simulink model "Bouclage_L"  (R2018b)
settings: Solver=ode45  StartTime=0.0  StopTime=10.0  RelTol=1e-4  EnableMultiTasking=on
values from neighbouring files (symbols this model uses):
  A_nl = [0  0                    1                  0 ;            0  0                    0                  1 ;            0  Ks/Jp                -Phi^2*N^2/(R*Jp)  0 ;            0  -Ks*(Jp+Jb)/(Jp*Jb)  Phi^2*N^2/(R*Jp)   0]    [Script_TP1.m]
  B_nl = [B B_b]    [Script_TP1.m]
  beta = R*Jp*Jb/(Ks*N*Phi)    (= 3.72670807453e-05)    [Script_TP1.m]
  C = [1,  1,  0,  0]    [Script_TP1.m]
  Jb = 0.0059    [Script_TP1.m]
  Ks = 1.61    [Script_TP1.m]
  L = [0, -Ks^2*(Jp+Jb)/(Jp*Jb^2) , Ks*Phi^2*N^2/(R*Jp*Jb), 0]    [Script_TP1.m]
  l1 = m*g*h/Jb    (= 40.1633898305)    [Script_TP1.m]
  l2 = -(m*g*h)^2/(Jb*Jb)    (= -1613.09788268)    [Script_TP1.m]
  l3 = Ks*m*g*h/(Jb^2)    (= 10959.8402758)    [Script_TP1.m]
  l4 = Ks*m*g*h/(Jb*Jb)    (= 10959.8402758)    [Script_TP1.m]
  Somme = [1 1 1 1 1]    [Script_TP1.m]
libraries: simulink x1
settings Model: Creator=abbasturki  LastModifiedBy=pac
settings DataIOCC: LimitDataPoints=on  SaveFormat=Array
settings OptimizationCC: ExpressionDepthLimit=2147483647  LifeSpan=inf
settings DebuggingCC: UnderspecifiedInitializationDetection=Classic  MergeDetectMultiDrivingBlocksExec=none  SolverPrmCheckMsg=warning  StateNameClashWarn=warning  SFUnexpectedBacktrackingDiag=warning  SFNoUnconditionalDefaultTransitionDiag=warning  SFExecutionAtInitializationDiag=none
settings HardwareCC: ProdBitPerPointer=32  ProdBitPerSizeT=32  ProdBitPerPtrDiffT=32  ProdLargestAtomicFloat=None  ProdIntDivRoundTo=Undefined  ProdEndianess=Unspecified  ProdWordSize=32  ProdHWDeviceType=32-bit Generic
settings ModelReferenceCC: PropagateSignalLabelsOutOfModel=off
settings SFSimCC: SimUseLocalCustomCode=off
settings RTWCC: RTWUseLocalCustomCode=off
settings CodeAppCC: StateflowObjectComments=on
settings GRTTargetCC: TargetLangStandard=C89/C90 (ANSI)  GeneratePreprocessorConditionals=Disable all  CombineOutputUpdateFcns=off  GRTInterface=on
settings ConfigComp: CovMetricSettings=dw  CovHtmlReporting=on  CovSaveCumulativeToWorkspaceVar=on  CovSaveSingleToWorkspaceVar=on  CovExternalEMLEnable=off

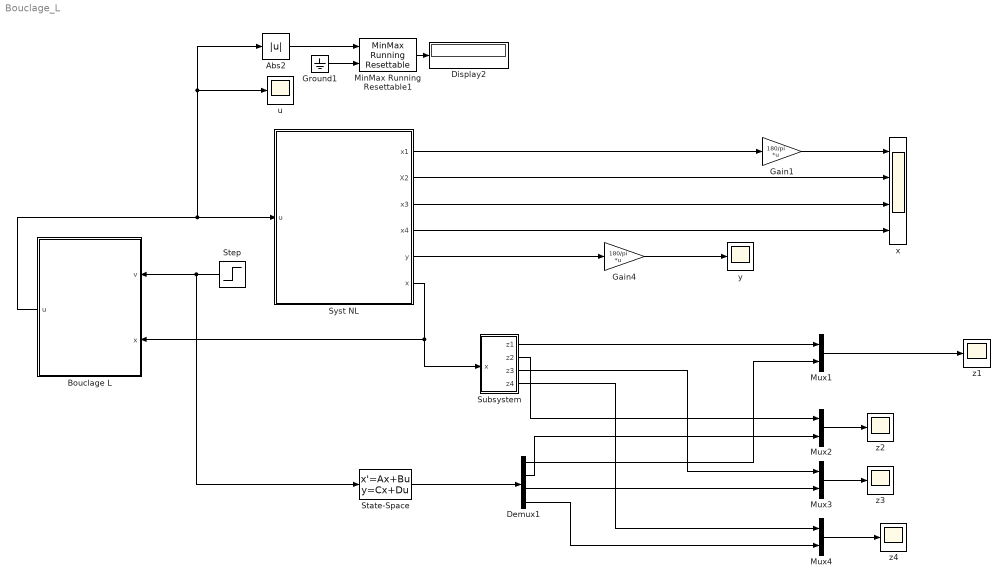
== system Bouclage_L ==
  Abs2 : Abs
  Bouclage L : Subsystem
  Demux1 : Demux
  Display2 : Display
  Gain1 : Gain  Gain=180/pi  Multiplication=Matrix(K*u)
  Gain4 : Gain  Gain=180/pi  Multiplication=Matrix(K*u)
  Ground1 : Ground
  MinMax Running Resettable1 : simulink/Math Operations/MinMax Running Resettable  Function=max  vinit=0.0
  Mux{1..4} (4 alike) : Mux  Inputs=2
  State-Space : StateSpace  A=[0 1 0 0; 0 0 1 0; 0 0 0 1; 0 0 0 0]  B=[0;0;0;1]  C=eye(4)  D=zeros(4,1)  InitialCondition=0
  Step : Step  Time=0  SampleTime=0
  Subsystem : Subsystem
  Syst NL : Subsystem
  u : Scope
  x : Scope  NumInputPorts=4
  y : Scope
  z{1..4} (4 alike) : Scope
  wires:
  Syst NL/3(x3) -> x/3
  Syst NL/4(x4) -> x/4
  Bouclage L/1(u) -> u/1, Abs2/1, Syst NL/1(u)
  Abs2/1 -> MinMax Running Resettable1/1
  MinMax Running Resettable1/1 -> Display2/1
  Ground1/1 -> MinMax Running Resettable1/2
  Syst NL/1(x1) -> Gain1/1
  Syst NL/5(y) -> Gain4/1
  Syst NL/2(X2) -> x/2
  Gain1/1 -> x/1
  Gain4/1 -> y/1
  Syst NL/6(x) -> Subsystem/1(x), Bouclage L/2(x)
  Step/1 -> State-Space/1, Bouclage L/1(v)
  State-Space/1 -> Demux1/1
  Subsystem/1(z1) -> Mux1/1
  Mux1/1 -> z1/1
  Mux2/1 -> z2/1
  Subsystem/2(z2) -> Mux2/1
  Demux1/2 -> Mux2/2
  Mux3/1 -> z3/1
  Subsystem/3(z3) -> Mux3/1
  Demux1/3 -> Mux3/2
  Mux4/1 -> z4/1
  Subsystem/4(z4) -> Mux4/1
  Demux1/4 -> Mux4/2
  Demux1/1 -> Mux1/2

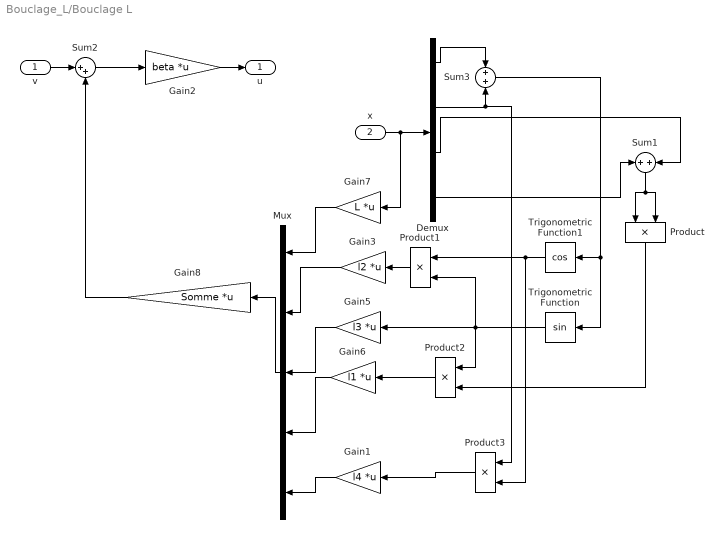
== system Bouclage_L/Bouclage L ==
  v : Inport
  x : Inport  Port=2
  Demux : Demux
  Gain1 : Gain  Gain=l4  Multiplication=Matrix(K*u)
  Gain2 : Gain  Gain=beta  Multiplication=Matrix(K*u)
  Gain3 : Gain  Gain=l2  Multiplication=Matrix(K*u)
  Gain5 : Gain  Gain=l3  Multiplication=Matrix(K*u)
  Gain6 : Gain  Gain=l1  Multiplication=Matrix(K*u)
  Gain7 : Gain  Gain=L  Multiplication=Matrix(K*u)
  Gain8 : Gain  Gain=Somme  Multiplication=Matrix(K*u)
  Mux : Mux  Inputs=5
  Product{,1..3} (4 alike) : Product  RndMeth=Zero
  Sum1 : Sum
  Sum2 : Sum  Inputs=|++
  Sum3 : Sum
  Trigonometric Function : Trigonometry
  Trigonometric Function1 : Trigonometry  Operator=cos
  u : Outport
  wires:
  Sum1/1 -> Product/1, Product/2
  Product1/1 -> Gain3/1
  Trigonometric Function1/1 -> Product1/1, Product3/2
  Trigonometric Function/1 -> Product1/2, Gain5/1, Product2/1
  Product/1 -> Product2/2
  Product2/1 -> Gain6/1
  Mux/1 -> Gain8/1
  Gain6/1 -> Mux/4
  Gain5/1 -> Mux/3
  Gain3/1 -> Mux/2
  Gain7/1 -> Mux/1
  Sum2/1 -> Gain2/1
  Gain8/1 -> Sum2/2
  Demux/4 -> Sum1/1
  Demux/3 -> Sum1/2
  Sum3/1 -> Trigonometric Function1/1, Trigonometric Function/1
  Gain2/1 -> u/1
  v/1 -> Sum2/1
  x/1 -> Demux/1, Gain7/1
  Demux/1 -> Sum3/1
  Demux/2 -> Product3/1, Sum3/2
  Gain1/1 -> Mux/5
  Product3/1 -> Gain1/1

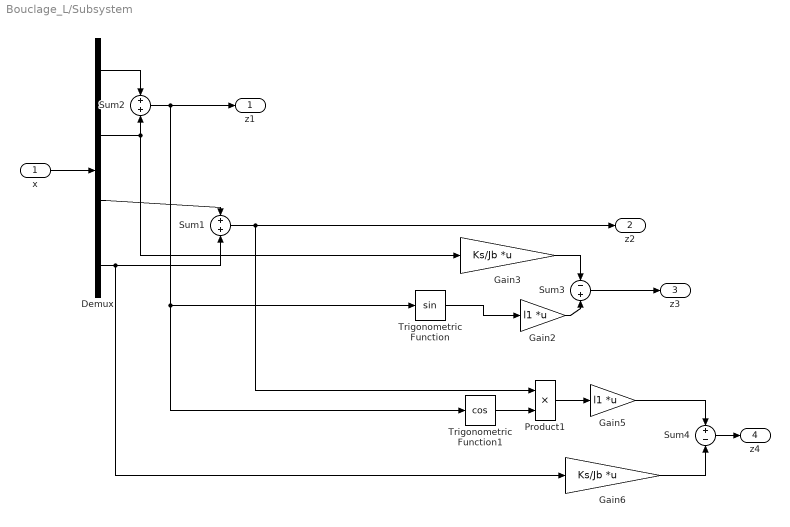
== system Bouclage_L/Subsystem ==
  x : Inport
  Demux : Demux
  Gain2 : Gain  Gain=l1  Multiplication=Matrix(K*u)
  Gain3 : Gain  Gain=Ks/Jb  Multiplication=Matrix(K*u)
  Gain5 : Gain  Gain=l1  Multiplication=Matrix(K*u)
  Gain6 : Gain  Gain=Ks/Jb  Multiplication=Matrix(K*u)
  Product1 : Product  RndMeth=Zero
  Sum1 : Sum
  Sum2 : Sum
  Sum3 : Sum  Inputs=-+
  Sum4 : Sum  Inputs=+-
  Trigonometric Function : Trigonometry
  Trigonometric Function1 : Trigonometry  Operator=cos
  z1 : Outport
  z2 : Outport  Port=2
  z3 : Outport  Port=3
  z4 : Outport  Port=4
  wires:
  Gain3/1 -> Sum3/1
  Trigonometric Function/1 -> Gain2/1
  Trigonometric Function1/1 -> Product1/2
  Product1/1 -> Gain5/1
  Gain6/1 -> Sum4/2
  Demux/4 -> Gain6/1, Sum1/2
  Sum4/1 -> z4/1
  Demux/2 -> Gain3/1, Sum2/2
  Demux/1 -> Sum2/1
  Sum2/1 -> Trigonometric Function1/1, Trigonometric Function/1, z1/1
  Demux/3 -> Sum1/1
  Sum1/1 -> z2/1, Product1/1
  x/1 -> Demux/1
  Gain5/1 -> Sum4/1
  Gain2/1 -> Sum3/2
  Sum3/1 -> z3/1

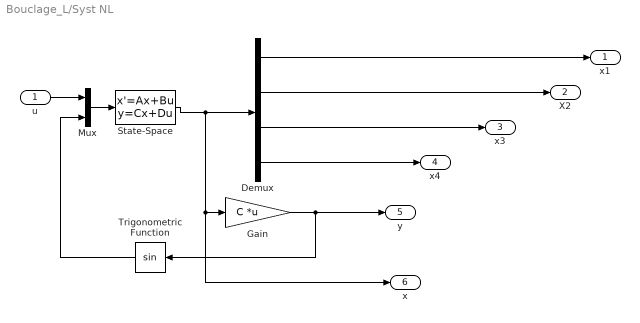
== system Bouclage_L/Syst NL ==
  u : Inport
  Demux : Demux
  Gain : Gain  Gain=C  Multiplication=Matrix(K*u)
  Mux : Mux  Inputs=2
  State-Space : StateSpace  A=A_nl  B=B_nl  C=eye(4)  D=zeros(4,2)  InitialCondition=0
  Trigonometric Function : Trigonometry
  x1 : Outport
  X2 : Outport  Port=2
  x3 : Outport  Port=3
  x4 : Outport  Port=4
  y : Outport  Port=5
  x : Outport  Port=6
  wires:
  State-Space/1 -> Demux/1, Gain/1, x/1
  Demux/1 -> x1/1
  Demux/2 -> X2/1
  Gain/1 -> y/1, Trigonometric Function/1
  Mux/1 -> State-Space/1
  Trigonometric Function/1 -> Mux/2
  u/1 -> Mux/1
  Demux/3 -> x3/1
  Demux/4 -> x4/1
